simulink model "twoaxisgimbal_trackingloop"  (R2023a)
settings: Solver=VariableStepAuto  StartTime=0.0  StopTime=100  RelTol=1e-3
libraries: slpidlib x4, simulink x2
settings Model: Creator=hazar  LastModifiedBy=hazar
settings SolverCC: MaxConsecutiveMinStep=10

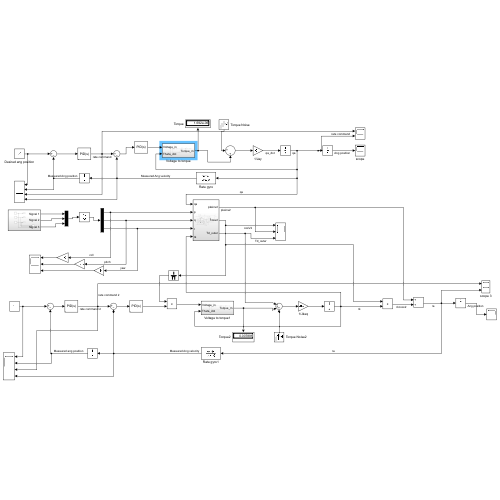
[thumbnail: Simulink's stored preview of the top-level diagram]
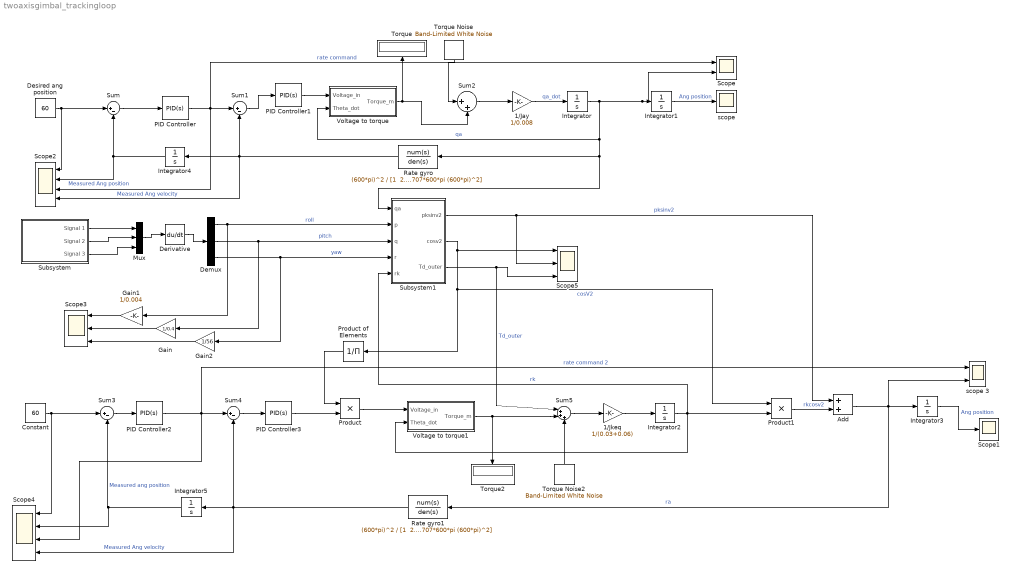
== system twoaxisgimbal_trackingloop ==
  1/Jay : Gain  Gain=1/0.008
  1/Jkeq : Gain  Gain=1/(0.03+0.06)
  Add : Sum
  Constant : Constant  Value=60
  Demux : Demux  Outputs=3
  Derivative : Derivative
  Desired ang position : Constant  Value=60
  Gain : Gain  Gain=1/0.4
  Gain1 : Gain  Gain=1/0.004
  Gain2 : Gain  Gain=1/56
  Integrator{,1..5} (6 alike) : Integrator
  Mux : Mux  Inputs=3
  PID Controller : slpidlib/PID Controller  Controller=PID  Form=Parallel  TimeDomain=Continuous-time  UseExternalTs=off  SampleTime=-1  IntegratorMethod=Forward Euler  FilterMethod=Forward Euler  ControllerParametersSource=internal  P=2.4942948626399  I=0.290538467638859  UseKiTs=off  D=0.373045797939572  N=142.16039231583  UseFilter=on  TunerSelectOption=Transfer Function Based (PID Tuner App)  InitialConditionSource=internal  InitialConditionForIntegrator=0  InitialConditionForFilter=0  DifferentiatorICPrevScaledInput=0  ExternalReset=none  TrackingMode=off  Kt=1  LimitOutput=off  SatLimitsSource=internal  UpperSaturationLimit=inf  LowerSaturationLimit=-inf  LinearizeAsGain=on  AntiWindupMode=none  Kb=1  LimitIntegrator=off  UpperIntegratorSaturationLimit=inf  LowerIntegratorSaturationLimit=-inf  POutMin=[]  POutMax=[]  IOutMin=[]  IOutMax=[]  DOutMin=[]  DOutMax=[]  NOutMin=[]  NOutMax=[]  SumOutMin=[]  SumOutMax=[]  SaturationOutMin=[]  SaturationOutMax=[]  PParamMin=[]  PParamMax=[]  IParamMin=[]  IParamMax=[]  DParamMin=[]  DParamMax=[]  NParamMin=[]  NParamMax=[]  KbParamMin=[]  KbParamMax=[]  KtParamMin=[]  KtParamMax=[]  KbOutMin=[]  KbOutMax=[]  KtOutMin=[]  KtOutMax=[]  IntegratorOutMin=[]  IntegratorOutMax=[]  FilterOutMin=[]  FilterOutMax=[]  SumI1OutMin=[]  SumI1OutMax=[]  SumI2OutMin=[]  SumI2OutMax=[]  SumI3OutMin=[]  SumI3OutMax=[]  SumI4OutMin=[]  SumI4OutMax=[]  SumDOutMin=[]  SumDOutMax=[]  DifferentiatorOutMin=[]  DifferentiatorOutMax=[]  FilterDiffOutCoefMin=[]  FilterDiffOutCoefMax=[]  ReciprocalOutMin=[]  ReciprocalOutMax=[]  SumDenOutMin=[]  SumDenOutMax=[]  SumNumOutMin=[]  SumNumOutMax=[]  DivideOutMin=[]  DivideOutMax=[]  UdiffTsProdOutMin=[]  UdiffTsProdOutMax=[]  NTsProdOutMin=[]  NTsProdOutMax=[]  UintegralTsProdOutMin=[]  UintegralTsProdOutMax=[]  UngainTsProdOutMin=[]  UngainTsProdOutMax=[]  ClampingZeroOutDataTypeStr=Inherit: Inherit via back propagation  ClampingZeroOutMin=[]  ClampingZeroOutMax=[]  FilterDenConstantOutDataTypeStr=Inherit: Inherit via back propagation  FilterDenConstantOutMin=[]  FilterDenConstantOutMax=[]  PCopyOutDataTypeStr=Inherit: Inherit via back propagation  PCopyOutMin=[]  PCopyOutMax=[]  NCopyOutDataTypeStr=Inherit: Inherit via back propagation  NCopyOutMin=[]  NCopyOutMax=[]  IntegratorContinuousStateAttributes=''  IntegratorStateMustResolveToSignalObject=off  IntegratorRTWStateStorageClass=Auto  FilterContinuousStateAttributes=''  FilterStateMustResolveToSignalObject=off  FilterRTWStateStorageClass=Auto  ParallelPVariant=InternalParameters  IdealPVariant=Disabled  IVariant=InternalParameters  DVariant=InternalParameters  IntegratorVariant=Continuous  SatVariant=Disabled  AWVariant=Passthrough  PCopyVariant=Disabled  TRVariant=Disabled  FdbkBlocksVariant=Forward  IdealPFdbkVariant=Disabled  SatFdbkVariant=Disabled  DerivativeFilterVariant=ContFilter  NVariant=InternalParameters  NCopyVariant=Disabled  FilterICVariant=InternalICsFilter  IntegratorICVariant=InternalICs  ExternalResetVariant=Disabled  TRSumVariant=Passthrough  SumFdbkVariant=Disabled  SumVariant=Sum_PID  TsampFilterVariant=InternalTs  TsampNgainVariant=Passthrough  TsampIntegralVariant=Disabled_SignalSpec  ExternalSaturationOutDataTypeStr=Inherit: Same as second input
  PID Controller1 : slpidlib/PID Controller  Controller=PID  Form=Parallel  TimeDomain=Continuous-time  UseExternalTs=off  SampleTime=-1  IntegratorMethod=Forward Euler  FilterMethod=Forward Euler  ControllerParametersSource=internal  P=0.184015245496125  I=0.00327855652286255  UseKiTs=off  D=-0.0947245304110595  N=1.9426356055563  UseFilter=on  TunerSelectOption=Transfer Function Based (PID Tuner App)  InitialConditionSource=internal  InitialConditionForIntegrator=0  InitialConditionForFilter=0  DifferentiatorICPrevScaledInput=0  ExternalReset=none  TrackingMode=off  Kt=1  LimitOutput=off  SatLimitsSource=internal  UpperSaturationLimit=inf  LowerSaturationLimit=-inf  LinearizeAsGain=on  AntiWindupMode=none  Kb=1  LimitIntegrator=off  UpperIntegratorSaturationLimit=inf  LowerIntegratorSaturationLimit=-inf  POutMin=[]  POutMax=[]  IOutMin=[]  IOutMax=[]  DOutMin=[]  DOutMax=[]  NOutMin=[]  NOutMax=[]  SumOutMin=[]  SumOutMax=[]  SaturationOutMin=[]  SaturationOutMax=[]  PParamMin=[]  PParamMax=[]  IParamMin=[]  IParamMax=[]  DParamMin=[]  DParamMax=[]  NParamMin=[]  NParamMax=[]  KbParamMin=[]  KbParamMax=[]  KtParamMin=[]  KtParamMax=[]  KbOutMin=[]  KbOutMax=[]  KtOutMin=[]  KtOutMax=[]  IntegratorOutMin=[]  IntegratorOutMax=[]  FilterOutMin=[]  FilterOutMax=[]  SumI1OutMin=[]  SumI1OutMax=[]  SumI2OutMin=[]  SumI2OutMax=[]  SumI3OutMin=[]  SumI3OutMax=[]  SumI4OutMin=[]  SumI4OutMax=[]  SumDOutMin=[]  SumDOutMax=[]  DifferentiatorOutMin=[]  DifferentiatorOutMax=[]  FilterDiffOutCoefMin=[]  FilterDiffOutCoefMax=[]  ReciprocalOutMin=[]  ReciprocalOutMax=[]  SumDenOutMin=[]  SumDenOutMax=[]  SumNumOutMin=[]  SumNumOutMax=[]  DivideOutMin=[]  DivideOutMax=[]  UdiffTsProdOutMin=[]  UdiffTsProdOutMax=[]  NTsProdOutMin=[]  NTsProdOutMax=[]  UintegralTsProdOutMin=[]  UintegralTsProdOutMax=[]  UngainTsProdOutMin=[]  UngainTsProdOutMax=[]  ClampingZeroOutDataTypeStr=Inherit: Inherit via back propagation  ClampingZeroOutMin=[]  ClampingZeroOutMax=[]  FilterDenConstantOutDataTypeStr=Inherit: Inherit via back propagation  FilterDenConstantOutMin=[]  FilterDenConstantOutMax=[]  PCopyOutDataTypeStr=Inherit: Inherit via back propagation  PCopyOutMin=[]  PCopyOutMax=[]  NCopyOutDataTypeStr=Inherit: Inherit via back propagation  NCopyOutMin=[]  NCopyOutMax=[]  IntegratorContinuousStateAttributes=''  IntegratorStateMustResolveToSignalObject=off  IntegratorRTWStateStorageClass=Auto  FilterContinuousStateAttributes=''  FilterStateMustResolveToSignalObject=off  FilterRTWStateStorageClass=Auto  ParallelPVariant=InternalParameters  IdealPVariant=Disabled  IVariant=InternalParameters  DVariant=InternalParameters  IntegratorVariant=Continuous  SatVariant=Disabled  AWVariant=Passthrough  PCopyVariant=Disabled  TRVariant=Disabled  FdbkBlocksVariant=Forward  IdealPFdbkVariant=Disabled  SatFdbkVariant=Disabled  DerivativeFilterVariant=ContFilter  NVariant=InternalParameters  NCopyVariant=Disabled  FilterICVariant=InternalICsFilter  IntegratorICVariant=InternalICs  ExternalResetVariant=Disabled  TRSumVariant=Passthrough  SumFdbkVariant=Disabled  SumVariant=Sum_PID  TsampFilterVariant=InternalTs  TsampNgainVariant=Passthrough  TsampIntegralVariant=Disabled_SignalSpec  ExternalSaturationOutDataTypeStr=Inherit: Same as second input
  PID Controller2 : slpidlib/PID Controller  Controller=PID  Form=Parallel  TimeDomain=Continuous-time  UseExternalTs=off  SampleTime=-1  IntegratorMethod=Forward Euler  FilterMethod=Forward Euler  ControllerParametersSource=internal  P=0.301803944122495  I=0.00767644411223917  UseKiTs=off  D=1.52097449829221  N=2.307783846622  UseFilter=on  TunerSelectOption=Transfer Function Based (PID Tuner App)  InitialConditionSource=internal  InitialConditionForIntegrator=0  InitialConditionForFilter=0  DifferentiatorICPrevScaledInput=0  ExternalReset=none  TrackingMode=off  Kt=1  LimitOutput=off  SatLimitsSource=internal  UpperSaturationLimit=inf  LowerSaturationLimit=-inf  LinearizeAsGain=on  AntiWindupMode=none  Kb=1  LimitIntegrator=off  UpperIntegratorSaturationLimit=inf  LowerIntegratorSaturationLimit=-inf  POutMin=[]  POutMax=[]  IOutMin=[]  IOutMax=[]  DOutMin=[]  DOutMax=[]  NOutMin=[]  NOutMax=[]  SumOutMin=[]  SumOutMax=[]  SaturationOutMin=[]  SaturationOutMax=[]  PParamMin=[]  PParamMax=[]  IParamMin=[]  IParamMax=[]  DParamMin=[]  DParamMax=[]  NParamMin=[]  NParamMax=[]  KbParamMin=[]  KbParamMax=[]  KtParamMin=[]  KtParamMax=[]  KbOutMin=[]  KbOutMax=[]  KtOutMin=[]  KtOutMax=[]  IntegratorOutMin=[]  IntegratorOutMax=[]  FilterOutMin=[]  FilterOutMax=[]  SumI1OutMin=[]  SumI1OutMax=[]  SumI2OutMin=[]  SumI2OutMax=[]  SumI3OutMin=[]  SumI3OutMax=[]  SumI4OutMin=[]  SumI4OutMax=[]  SumDOutMin=[]  SumDOutMax=[]  DifferentiatorOutMin=[]  DifferentiatorOutMax=[]  FilterDiffOutCoefMin=[]  FilterDiffOutCoefMax=[]  ReciprocalOutMin=[]  ReciprocalOutMax=[]  SumDenOutMin=[]  SumDenOutMax=[]  SumNumOutMin=[]  SumNumOutMax=[]  DivideOutMin=[]  DivideOutMax=[]  UdiffTsProdOutMin=[]  UdiffTsProdOutMax=[]  NTsProdOutMin=[]  NTsProdOutMax=[]  UintegralTsProdOutMin=[]  UintegralTsProdOutMax=[]  UngainTsProdOutMin=[]  UngainTsProdOutMax=[]  ClampingZeroOutDataTypeStr=Inherit: Inherit via back propagation  ClampingZeroOutMin=[]  ClampingZeroOutMax=[]  FilterDenConstantOutDataTypeStr=Inherit: Inherit via back propagation  FilterDenConstantOutMin=[]  FilterDenConstantOutMax=[]  PCopyOutDataTypeStr=Inherit: Inherit via back propagation  PCopyOutMin=[]  PCopyOutMax=[]  NCopyOutDataTypeStr=Inherit: Inherit via back propagation  NCopyOutMin=[]  NCopyOutMax=[]  IntegratorContinuousStateAttributes=''  IntegratorStateMustResolveToSignalObject=off  IntegratorRTWStateStorageClass=Auto  FilterContinuousStateAttributes=''  FilterStateMustResolveToSignalObject=off  FilterRTWStateStorageClass=Auto  ParallelPVariant=InternalParameters  IdealPVariant=Disabled  IVariant=InternalParameters  DVariant=InternalParameters  IntegratorVariant=Continuous  SatVariant=Disabled  AWVariant=Passthrough  PCopyVariant=Disabled  TRVariant=Disabled  FdbkBlocksVariant=Forward  IdealPFdbkVariant=Disabled  SatFdbkVariant=Disabled  DerivativeFilterVariant=ContFilter  NVariant=InternalParameters  NCopyVariant=Disabled  FilterICVariant=InternalICsFilter  IntegratorICVariant=InternalICs  ExternalResetVariant=Disabled  TRSumVariant=Passthrough  SumFdbkVariant=Disabled  SumVariant=Sum_PID  TsampFilterVariant=InternalTs  TsampNgainVariant=Passthrough  TsampIntegralVariant=Disabled_SignalSpec  ExternalSaturationOutDataTypeStr=Inherit: Same as second input
  PID Controller3 : slpidlib/PID Controller  Controller=PID  Form=Parallel  TimeDomain=Continuous-time  UseExternalTs=off  SampleTime=-1  IntegratorMethod=Forward Euler  FilterMethod=Forward Euler  ControllerParametersSource=internal  P=0.390517044296606  I=0.00909392035675338  UseKiTs=off  D=-1.76715907196503  N=0.220985790408988  UseFilter=on  TunerSelectOption=Transfer Function Based (PID Tuner App)  InitialConditionSource=internal  InitialConditionForIntegrator=0  InitialConditionForFilter=0  DifferentiatorICPrevScaledInput=0  ExternalReset=none  TrackingMode=off  Kt=1  LimitOutput=off  SatLimitsSource=internal  UpperSaturationLimit=inf  LowerSaturationLimit=-inf  LinearizeAsGain=on  AntiWindupMode=none  Kb=1  LimitIntegrator=off  UpperIntegratorSaturationLimit=inf  LowerIntegratorSaturationLimit=-inf  POutMin=[]  POutMax=[]  IOutMin=[]  IOutMax=[]  DOutMin=[]  DOutMax=[]  NOutMin=[]  NOutMax=[]  SumOutMin=[]  SumOutMax=[]  SaturationOutMin=[]  SaturationOutMax=[]  PParamMin=[]  PParamMax=[]  IParamMin=[]  IParamMax=[]  DParamMin=[]  DParamMax=[]  NParamMin=[]  NParamMax=[]  KbParamMin=[]  KbParamMax=[]  KtParamMin=[]  KtParamMax=[]  KbOutMin=[]  KbOutMax=[]  KtOutMin=[]  KtOutMax=[]  IntegratorOutMin=[]  IntegratorOutMax=[]  FilterOutMin=[]  FilterOutMax=[]  SumI1OutMin=[]  SumI1OutMax=[]  SumI2OutMin=[]  SumI2OutMax=[]  SumI3OutMin=[]  SumI3OutMax=[]  SumI4OutMin=[]  SumI4OutMax=[]  SumDOutMin=[]  SumDOutMax=[]  DifferentiatorOutMin=[]  DifferentiatorOutMax=[]  FilterDiffOutCoefMin=[]  FilterDiffOutCoefMax=[]  ReciprocalOutMin=[]  ReciprocalOutMax=[]  SumDenOutMin=[]  SumDenOutMax=[]  SumNumOutMin=[]  SumNumOutMax=[]  DivideOutMin=[]  DivideOutMax=[]  UdiffTsProdOutMin=[]  UdiffTsProdOutMax=[]  NTsProdOutMin=[]  NTsProdOutMax=[]  UintegralTsProdOutMin=[]  UintegralTsProdOutMax=[]  UngainTsProdOutMin=[]  UngainTsProdOutMax=[]  ClampingZeroOutDataTypeStr=Inherit: Inherit via back propagation  ClampingZeroOutMin=[]  ClampingZeroOutMax=[]  FilterDenConstantOutDataTypeStr=Inherit: Inherit via back propagation  FilterDenConstantOutMin=[]  FilterDenConstantOutMax=[]  PCopyOutDataTypeStr=Inherit: Inherit via back propagation  PCopyOutMin=[]  PCopyOutMax=[]  NCopyOutDataTypeStr=Inherit: Inherit via back propagation  NCopyOutMin=[]  NCopyOutMax=[]  IntegratorContinuousStateAttributes=''  IntegratorStateMustResolveToSignalObject=off  IntegratorRTWStateStorageClass=Auto  FilterContinuousStateAttributes=''  FilterStateMustResolveToSignalObject=off  FilterRTWStateStorageClass=Auto  ParallelPVariant=InternalParameters  IdealPVariant=Disabled  IVariant=InternalParameters  DVariant=InternalParameters  IntegratorVariant=Continuous  SatVariant=Disabled  AWVariant=Passthrough  PCopyVariant=Disabled  TRVariant=Disabled  FdbkBlocksVariant=Forward  IdealPFdbkVariant=Disabled  SatFdbkVariant=Disabled  DerivativeFilterVariant=ContFilter  NVariant=InternalParameters  NCopyVariant=Disabled  FilterICVariant=InternalICsFilter  IntegratorICVariant=InternalICs  ExternalResetVariant=Disabled  TRSumVariant=Passthrough  SumFdbkVariant=Disabled  SumVariant=Sum_PID  TsampFilterVariant=InternalTs  TsampNgainVariant=Passthrough  TsampIntegralVariant=Disabled_SignalSpec  ExternalSaturationOutDataTypeStr=Inherit: Same as second input
  Product : Product
  Product of Elements : Product  Inputs=/
  Product1 : Product
  Rate gyro : TransferFcn  Numerator=(600*pi)^2  Denominator="[1  2*0.707*600*pi (600*pi)^2]"
  Rate gyro1 : TransferFcn  Numerator=(600*pi)^2  Denominator="[1  2*0.707*600*pi (600*pi)^2]"
  Scope : Scope  NumInputPorts=2
  Scope1 : Scope
  Scope2 : Scope  NumInputPorts=4
  Scope3 : Scope  NumInputPorts=3
  Scope4 : Scope  NumInputPorts=4
  Scope5 : Scope  NumInputPorts=3
  Subsystem : Subsystem
  Subsystem1 : Subsystem
  Sum{,1,3..4} (4 alike) : Sum  Inputs=|+-
  Sum2 : Sum  Inputs=|++
  Sum5 : Sum  Inputs=|+++
  Torque : Display
  Torque Noise : simulink/Sources/Band-Limited White Noise  Cov=[0.00000000000022]  Ts=0.1  seed=[23341]
  Torque Noise2 : simulink/Sources/Band-Limited White Noise  Cov=[0.00000000000022]  Ts=0.1  seed=[23341]
  Torque2 : Display
  Voltage to torque : Subsystem
  Voltage to torque1 : Subsystem
  scope : Scope
  scope 3 : Scope  NumInputPorts=2
  wires:
  Sum/1 -> PID Controller/1
  Sum1/1 -> PID Controller1/1
  PID Controller1/1 -> Voltage to torque/1(Voltage_in)
  Torque Noise/1 -> Sum2/1
  Sum2/1 -> 1/Jay/1
  1/Jay/1 -> Integrator/1  "qa_dot"
  1/Jkeq/1 -> Integrator2/1
  Add/1 -> Rate gyro1/1, Integrator3/1, scope 3/2  "ra"
  Integrator3/1 -> Scope1/1  "Ang position"
  Product1/1 -> Add/2  "rkcosv2"
  Derivative/1 -> Demux/1
  Demux/2 -> Gain/1, Subsystem1/3(q)  "pitch"
  Subsystem/2(Signal 2) -> Mux/2
  Subsystem/1(Signal 1) -> Mux/1
  Subsystem/3(Signal 3) -> Mux/3
  Mux/1 -> Derivative/1
  Demux/3 -> Gain2/1, Subsystem1/4(r)  "yaw"
  Subsystem1/2(cosv2) -> Product1/1, Product of Elements/1, Scope5/1  "cosV2"
  Integrator2/1 -> Product1/2, Voltage to torque1/2(Theta_dot), Subsystem1/5(rk)  "rk"
  Voltage to torque/1(Torque_m) -> Sum2/2, Torque/1
  Integrator1/1 -> scope/1  "Ang position"
  Demux/1 -> Gain1/1, Subsystem1/2(p)  "roll"
  Product of Elements/1 -> Product/1
  Product/1 -> Voltage to torque1/1(Voltage_in)
  Voltage to torque1/1(Torque_m) -> Sum5/2, Torque2/1
  Torque Noise2/1 -> Sum5/3
  Sum5/1 -> 1/Jkeq/1
  Integrator/1 -> Rate gyro/1, Subsystem1/1(qa), Voltage to torque/2(Theta_dot), Integrator1/1, Scope/2  "qa"
  Subsystem1/1(pksinv2) -> Scope5/2, Add/1  "pksinv2"
  PID Controller/1 -> Scope/1, Sum1/1, Scope2/3  "rate command"
  Desired ang position/1 -> Sum/1, Scope2/1
  Rate gyro/1 -> Scope2/4, Integrator4/1, Sum1/2  "Measured Ang velocity"
  Integrator4/1 -> Scope2/2, Sum/2  "Measured Ang position"
  Constant/1 -> Scope4/1, Sum3/1
  Integrator5/1 -> Scope4/2, Sum3/2  "Measured ang position"
  PID Controller2/1 -> scope 3/1, Sum4/1, Scope4/3  "rate command 2"
  Sum3/1 -> PID Controller2/1
  PID Controller3/1 -> Product/2
  Sum4/1 -> PID Controller3/1
  Subsystem1/3(Td_outer) -> Sum5/1, Scope5/3  "Td_outer"
  Rate gyro1/1 -> Sum4/2, Integrator5/1, Scope4/4  "Measured Ang velocity"
  Gain1/1 -> Scope3/1
  Gain/1 -> Scope3/2
  Gain2/1 -> Scope3/3

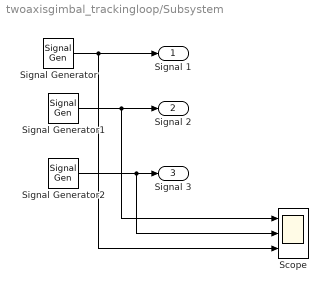
== system twoaxisgimbal_trackingloop/Subsystem ==
  Scope : Scope  NumInputPorts=3
  Signal Generator : SignalGenerator  Amplitude=2  Frequency=1/30
  Signal Generator1 : SignalGenerator  Amplitude=5  Frequency=1/25
  Signal Generator2 : SignalGenerator  Amplitude=3  Frequency=1/40
  Signal 1 : Outport
  Signal 2 : Outport  Port=2
  Signal 3 : Outport  Port=3
  wires:
  Signal Generator/1 -> Scope/3, Signal 1/1
  Signal Generator1/1 -> Signal 2/1, Scope/1
  Signal Generator2/1 -> Signal 3/1, Scope/2

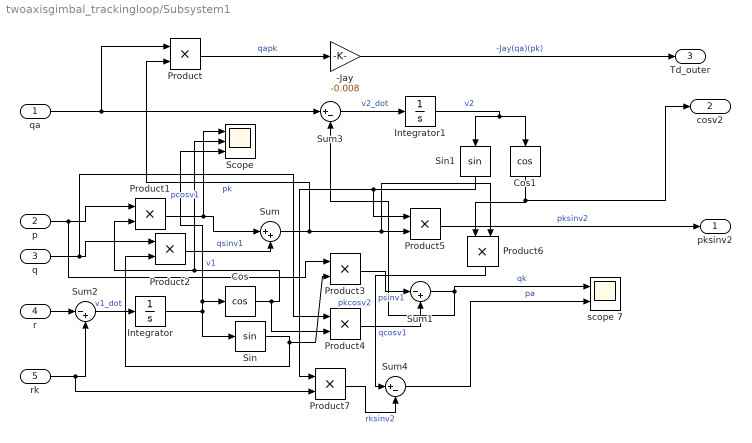
== system twoaxisgimbal_trackingloop/Subsystem1 ==
  qa : Inport
  p : Inport  Port=2
  q : Inport  Port=3
  r : Inport  Port=4
  rk : Inport  Port=5
  -Jay : Gain  Gain=-0.008
  Cos : Trigonometry  Operator=cos
  Cos1 : Trigonometry  Operator=cos
  Integrator : Integrator
  Integrator1 : Integrator
  Product{,1..7} (8 alike) : Product
  Scope : Scope  NumInputPorts=3
  Sin : Trigonometry
  Sin1 : Trigonometry
  Sum : Sum  Inputs=|++
  Sum1 : Sum  Inputs=|-+
  Sum2 : Sum  Inputs=|-+
  Sum3 : Sum  Inputs=|+-
  Sum4 : Sum  Inputs=|+-
  scope 7 : Scope  NumInputPorts=2
  pksinv2 : Outport
  cosv2 : Outport  Port=2
  Td_outer : Outport  Port=3
  wires:
  Sum2/1 -> Integrator/1  "v1_dot"
  Sin/1 -> Product3/2, Product2/2
  Cos/1 -> Product4/2, Scope/2, Product1/2
  Product5/1 -> pksinv2/1  "pksinv2"
  Product3/1 -> Sum1/1  "psinv1"
  Sin1/1 -> Product7/1, Product5/1
  q/1 -> Product4/1, Product2/1
  Product6/1 -> Sum4/1  "pkcosv2"
  Sum/1 -> Product/2, Product6/2, Product5/2  "pk"
  Integrator/1 -> Cos/1, Scope/3, Sin/1  "v1"
  Cos1/1 -> Product6/1, cosv2/1
  Product2/1 -> Sum/2  "qsinv1"
  Sum3/1 -> Integrator1/1  "v2_dot"
  p/1 -> Product3/1, Product1/1
  Product1/1 -> Scope/1, Sum/1  "pcosv1"
  Product7/1 -> Sum4/2  "rksinv2"
  Sum1/1 -> Sum3/2, scope 7/1  "qk"
  Product4/1 -> Sum1/2  "qcosv1"
  r/1 -> Sum2/1
  Sum4/1 -> scope 7/2  "pa"
  Integrator1/1 -> Cos1/1, Sin1/1  "v2"
  qa/1 -> Product/1, Sum3/1
  rk/1 -> Product7/2, Sum2/2
  Product/1 -> -Jay/1  "qapk"
  -Jay/1 -> Td_outer/1  "-Jay(qa)(pk)"

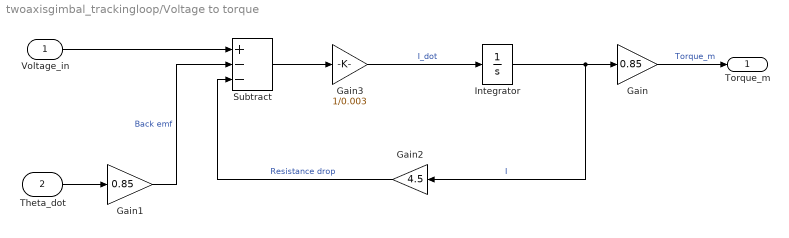
== system twoaxisgimbal_trackingloop/Voltage to torque ==
  Voltage_in : Inport
  Theta_dot : Inport  Port=2
  Gain : Gain  Gain=0.85
  Gain1 : Gain  Gain=0.85
  Gain2 : Gain  Gain=4.5
  Gain3 : Gain  Gain=1/0.003
  Integrator : Integrator
  Subtract : Sum  Inputs=+--
  Torque_m : Outport  VectorParamsAs1DForOutWhenUnconnected=off
  wires:
  Gain1/1 -> Subtract/2  "Back emf"
  Integrator/1 -> Gain2/1, Gain/1  "I"
  Subtract/1 -> Gain3/1
  Theta_dot/1 -> Gain1/1
  Gain3/1 -> Integrator/1  "I_dot"
  Gain/1 -> Torque_m/1  "Torque_m"
  Voltage_in/1 -> Subtract/1
  Gain2/1 -> Subtract/3  "Resistance drop"

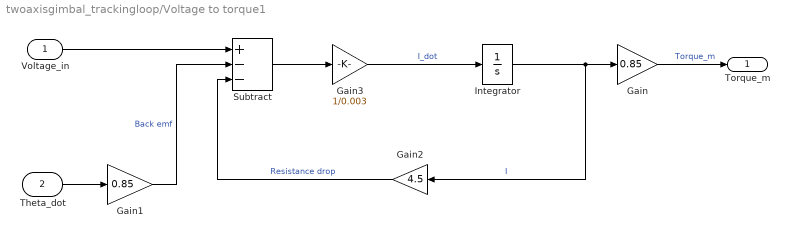
== system twoaxisgimbal_trackingloop/Voltage to torque1 ==
  Voltage_in : Inport
  Theta_dot : Inport  Port=2
  Gain : Gain  Gain=0.85
  Gain1 : Gain  Gain=0.85
  Gain2 : Gain  Gain=4.5
  Gain3 : Gain  Gain=1/0.003
  Integrator : Integrator
  Subtract : Sum  Inputs=+--
  Torque_m : Outport  VectorParamsAs1DForOutWhenUnconnected=off
  wires:
  Gain1/1 -> Subtract/2  "Back emf"
  Integrator/1 -> Gain2/1, Gain/1  "I"
  Subtract/1 -> Gain3/1
  Theta_dot/1 -> Gain1/1
  Gain3/1 -> Integrator/1  "I_dot"
  Gain/1 -> Torque_m/1  "Torque_m"
  Voltage_in/1 -> Subtract/1
  Gain2/1 -> Subtract/3  "Resistance drop"
